simulink model "pmdc_speed_control"  (R2023a)
settings: Solver=FixedStepAuto  StartTime=0.0  StopTime=1.2  FixedStep=1e-5  RelTol=1e-3
values from neighbouring files (symbols this model uses):
  B = 0    [parabtl.m]    (also in pmdc_parameter.m; testpara.m)
  IaN = 62    [parabtl.m]    (also in pmdc_parameter.m = 25; testpara.m = 25)
  J = 0.05    [dcmotor_parameter.m]    (also in parabtl.m; pmdc_parameter.m = 0.00252; testpara.m = 0.00252)
  KE = (Ua - Ra*Ia)*9.55/n    (= 1.17113806452)    [dcmotor_parameter.m]    (also in parabtl.m; pmdc_parameter.m = 0.424975; testpara.m = 0.424975)
  Ki = Kp/Ti    [parabtl.m]    (also in pmdc_parameter.m)
  Kiv = Kpv/Tiv    [parabtl.m]    (also in pmdc_parameter.m)
  Kp = (Ra*Ta*OmegaN)/(2*Zeta)    [parabtl.m]    (also in pmdc_parameter.m)
  Kpv = TMech/(2*Teq)    [parabtl.m]    (also in pmdc_parameter.m)
  KT = KE    (= 1.17113806452)    [dcmotor_parameter.m]    (also in parabtl.m; pmdc_parameter.m = 0.424975; testpara.m = 0.424975)
  La = 5.2e-3    (= 0.0052)    [dcmotor_parameter.m]    (also in parabtl.m; pmdc_parameter.m = 0.0017; testpara.m = 0.0017)
  Ra = 0.32    [dcmotor_parameter.m]    (also in parabtl.m; pmdc_parameter.m = 0.26; testpara.m = 0.26)
  Td = 1/fsw    (= 0.0002)    [parabtl.m]    (also in pmdc_parameter.m)
  Tfi = 1/(5*fsw)    (= 4e-05)    [parabtl.m]    (also in pmdc_parameter.m)
  Tfv = 5*Tfi    (= 0.0002)    [parabtl.m]    (also in pmdc_parameter.m)
  UaN = 400    [parabtl.m]    (also in pmdc_parameter.m = 140; testpara.m = 140)
libraries: spsMosfetLib x12, spsDCVoltageSourceLib x3, simulink x3, spsVoltageMeasurementLib x3, spsDCMachineLib x2, sps_lib x1
settings Model: Creator=luand  LastModifiedBy=luand

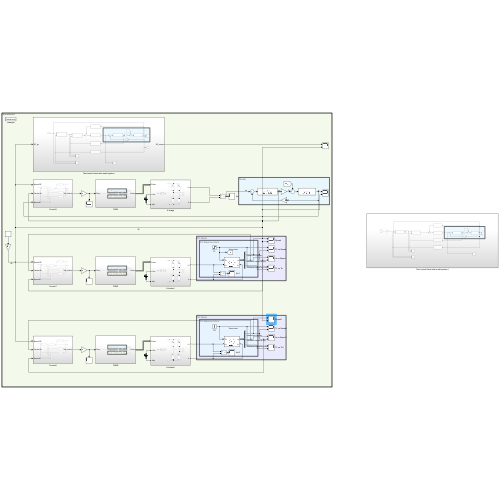
[thumbnail: Simulink's stored preview of the top-level diagram]
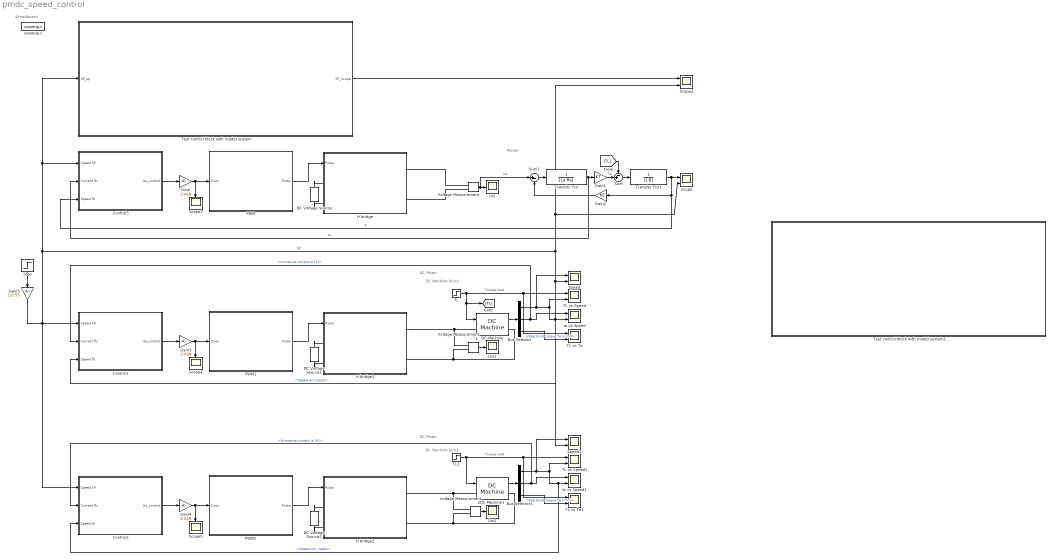
== system pmdc_speed_control ==
  note: Breadboard
  note: Model
  note: DC Motor
  note: DC Machine block
  note: DC Motor
  note: DC Machine block
  Bus Selector : BusSelector  OutputSignals=Speed wm (rad/s),Armature current ia (A),Electrical torque Te (n m)
  Bus Selector1 : BusSelector  OutputSignals=Speed wm (rad/s),Armature current ia (A),Electrical torque Te (n m)
  Control1 : Subsystem
  Control2 : Subsystem
  Control3 : Subsystem
  DC Machine : spsDCMachineLib/DC Machine  PresetModel=No  MechanicalLoad=Torque TL  FieldType=Permanent magnet  ShowDetailedParameters=on  MeasurementBus=off  RLa=[ Ra La ]  RLf="[ 240  120]"  Laf=1.8  MachineConstant=Torque constant (N.m/A)  Ke=1.8  Kt=KT  J=J  Bm=0  Tf=0  w0=0  Ifinit=1  TsPowergui=0  TsBlock=-1
  DC Machine1 : spsDCMachineLib/DC Machine  PresetModel=No  MechanicalLoad=Torque TL  FieldType=Permanent magnet  ShowDetailedParameters=on  MeasurementBus=off  RLa=[ Ra La ]  RLf="[ 240  120]"  Laf=1.8  MachineConstant=Torque constant (N.m/A)  Ke=1.8  Kt=KT  J=J  Bm=0  Tf=0  w0=0  Ifinit=1  TsPowergui=0  TsBlock=-1
  DC Voltage Source : spsDCVoltageSourceLib/DC Voltage Source  Amplitude=UaN  Measurements=None
  DC Voltage Source1 : spsDCVoltageSourceLib/DC Voltage Source  Amplitude=UaN  Measurements=None
  DC Voltage Source2 : spsDCVoltageSourceLib/DC Voltage Source  Amplitude=UaN  Measurements=None
  Gain : Gain  Gain=1/UaN
  Gain1 : Gain  Gain=KT
  Gain2 : Gain  Gain=KE
  Gain3 : Gain  Gain=1/UaN
  Gain4 : Gain  Gain=1/UaN
  Gain5 : Gain  Gain=1/9.55
  H bridge : Subsystem
  H bridge1 : Subsystem
  H bridge2 : Subsystem
  Ia vs Speed : Scope  NumInputPorts=2
  Ia vs Speed1 : Scope  NumInputPorts=2
  PWM : Subsystem
  PWM1 : Subsystem
  PWM2 : Subsystem
  Scope : Scope  NumInputPorts=2
  Scope2 : Scope  NumInputPorts=2
  Scope3 : Scope
  Scope4 : Scope
  Scope5 : Scope
  Speed : Scope  NumInputPorts=2
  Speed1 : Scope  NumInputPorts=2
  Step : Step  Time=.2  After=3000  SampleTime=0
  Sum : Sum  Inputs=-+|
  Sum1 : Sum  Inputs=|+-
  TL : Step  Time=0.3  After=0  SampleTime=0
  TL vs Speed : Scope  NumInputPorts=2
  TL vs Speed1 : Scope  NumInputPorts=2
  TL vs Te : Scope  NumInputPorts=2
  TL vs Te1 : Scope  NumInputPorts=2
  TL1 : Step  Time=0.3  After=0  SampleTime=0
  Test control block with model system : Subsystem
  Test control block with model system1 : Subsystem
  Transfer Fcn : TransferFcn  Denominator=[La Ra]
  Transfer Fcn1 : TransferFcn  Denominator=[J B]
  Uin : Scope
  Uin1 : Scope
  Uin2 : Scope
  Voltage Measurement : spsVoltageMeasurementLib/Voltage Measurement  PhasorSimulation=off  OutputType=Complex  PSBequivalent=0
  Voltage Measurement1 : spsVoltageMeasurementLib/Voltage Measurement  PhasorSimulation=off  OutputType=Complex  PSBequivalent=0
  Voltage Measurement2 : spsVoltageMeasurementLib/Voltage Measurement  PhasorSimulation=off  OutputType=Complex  PSBequivalent=0
  powergui : sps_lib/powergui  Priority=1  SimulationMode=Continuous  SampleTime=50e-6  frequency=60  Iterations=50  frequencyindice=0  Pbase=100e6  ErrMax=1e-4  UnitsV=kV  UnitsW=MW  buscounter=0  FunctionMessages=off  echomessages=off  EnableUseOfTLC=off  CurrentSourceSwitches=off  DisableSnubberDevices=off  DisableRonSwitches=off  DisableVfSwitches=off  DisplayEquations=off  AutomaticDiscreteSolvers=off  SolverType=Tustin/Backward Euler (TBE)  Interpol=off  ExternalGateDelay=off  methode=off  Ts=100  x0status=blocks  SPID=on  SwTol=0  HookPort=off  NonlinearTolerance=1e-4  nMaxIteration=100  ContinueOnMaxIteration=off  RestoreLinks=warning  ResistiveCurrentMeasurement=off  Frange=[0:2:500]  Ylog=off  Xlog=on  ShowGrid=off  save=off  variable=ZData  structure=0  ZoomFFT=off  StartTime=0.0  cycles=1  DisplayStyle=1  fundamental=60  FreqAxis=off  MaxFrequency=1000  frequencyindicesteady=1  RmsSteady=1  display=off
  wires:
  DC Machine/1 -> Bus Selector/1
  Bus Selector/2 -> Ia vs Speed/1, Control1/2(Current fb)  "<Armature current ia (A)>"
  Bus Selector/3 -> TL vs Te/2  "<Electrical torque Te (n m)>"
  Bus Selector/1 -> Speed/1, TL vs Speed/2, Control1/3(Speed fb), Ia vs Speed/2  "<Speed wm (rad/s)>"
  TL/1 -> DC Machine/1, [TL], TL vs Te/1, TL vs Speed/1  "Torque load"
  Control3/1(Ua_control) -> Gain/1
  PWM/1(Pulse) -> H bridge/1(Pulse)
  Voltage Measurement1/1 -> Uin1/1
  Voltage Measurement2/1 -> Uin2/1
  TL1/1 -> TL vs Speed1/1, TL vs Te1/1, DC Machine1/1  "Torque load"
  Bus Selector1/1 -> Control2/3(Speed fb), Ia vs Speed1/2, TL vs Speed1/2, Speed1/1  "<Speed wm (rad/s)>"
  Bus Selector1/3 -> TL vs Te1/2  "<Electrical torque Te (n m)>"
  Bus Selector1/2 -> Control2/2(Current fb), Ia vs Speed1/1  "<Armature current ia (A)>"
  DC Machine1/1 -> Bus Selector1/1
  Transfer Fcn/1 -> Control3/2(Current fb), Gain1/1  "Ia"
  Sum/1 -> Transfer Fcn1/1
  Sum1/1 -> Transfer Fcn/1
  Transfer Fcn1/1 -> Gain2/1, Control3/3(Speed fb), Scope/1  "w"
  Gain1/1 -> Sum/2  "Te"
  [TL] -> Sum/1
  Gain2/1 -> Sum1/2
  Voltage Measurement/1 -> Sum1/1, Uin/1  "Ua"
  Control1/1(Ua_control) -> Gain3/1
  PWM2/1(Pulse) -> H bridge2/1(Pulse)
  PWM1/1(Pulse) -> H bridge1/1(Pulse)
  Gain3/1 -> PWM1/1(Duty), Scope4/1
  Step/1 -> Gain5/1
  Gain5/1 -> Scope2/2, Scope/2, Speed/2, Speed1/2, Test control block with model system/1(SP_sp), Control3/1(Speed SP), Control2/1(Speed SP), Control1/1(Speed SP)  "SP"
  Control2/1(Ua_control) -> Gain4/1
  Gain4/1 -> PWM2/1(Duty), Scope5/1
  Test control block with model system/1(SP_scope) -> Scope2/1
  Gain/1 -> Scope3/1, PWM/1(Duty)
  connections:
  Voltage Measurement2/LConn2 -- DC Machine1/RConn1 -- H bridge2/RConn2
  Voltage Measurement2/LConn1 -- H bridge2/RConn1 -- DC Machine1/LConn1
  Voltage Measurement1/LConn2 -- H bridge1/RConn2 -- DC Machine/RConn1
  DC Voltage Source/RConn1 -- H bridge/LConn1
  DC Voltage Source/LConn1 -- H bridge/LConn2
  DC Voltage Source1/LConn1 -- H bridge1/LConn2
  DC Voltage Source1/RConn1 -- H bridge1/LConn1
  DC Voltage Source2/RConn1 -- H bridge2/LConn1
  DC Voltage Source2/LConn1 -- H bridge2/LConn2
  H bridge1/RConn1 -- DC Machine/LConn1 -- Voltage Measurement1/LConn1
  Voltage Measurement/LConn1 -- H bridge/RConn1
  Voltage Measurement/LConn2 -- H bridge/RConn2

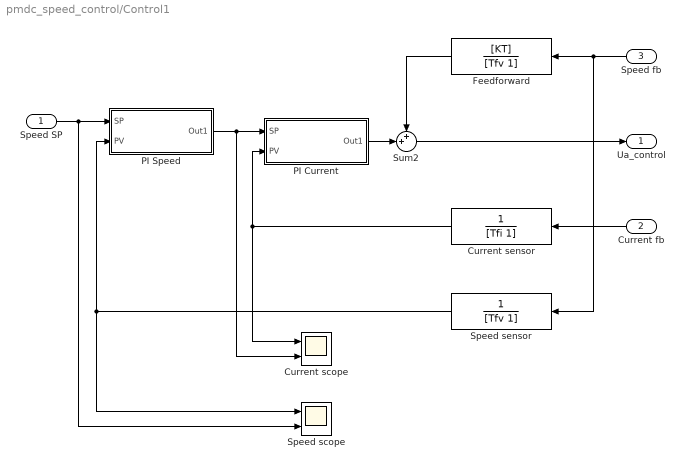
== system pmdc_speed_control/Control1 ==
  Speed SP : Inport
  Current fb : Inport  Port=2
  Speed fb : Inport  Port=3
  Current scope : Scope  NumInputPorts=2
  Current sensor : TransferFcn  Denominator=[Tfi 1]
  Feedforward : TransferFcn  Numerator=[KT]  Denominator=[Tfv 1]
  PI Current : Subsystem
  PI Speed : Subsystem
  Speed scope : Scope  NumInputPorts=2
  Speed sensor : TransferFcn  Denominator=[Tfv 1]
  Sum2 : Sum  Inputs=++|
  Ua_control : Outport
  wires:
  Speed SP/1 -> PI Speed/1(SP), Speed scope/2
  Speed sensor/1 -> Speed scope/1, PI Speed/2(PV)
  Sum2/1 -> Ua_control/1
  PI Current/1(Out1) -> Sum2/2
  Feedforward/1 -> Sum2/1
  Current sensor/1 -> PI Current/2(PV), Current scope/1
  PI Speed/1(Out1) -> PI Current/1(SP), Current scope/2
  Speed fb/1 -> Speed sensor/1, Feedforward/1
  Current fb/1 -> Current sensor/1

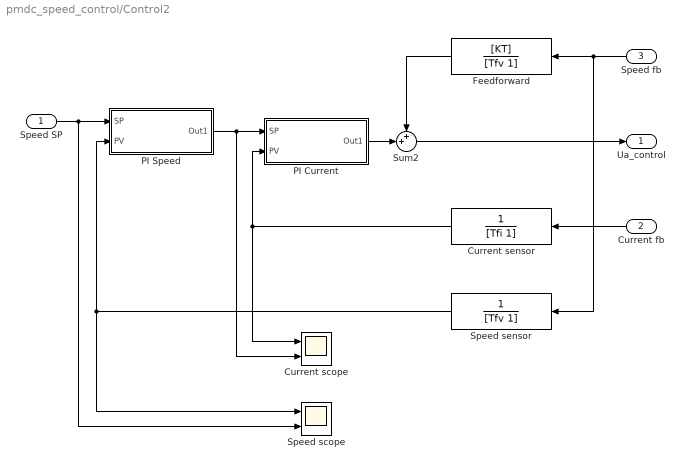
== system pmdc_speed_control/Control2 ==
  Speed SP : Inport
  Current fb : Inport  Port=2
  Speed fb : Inport  Port=3
  Current scope : Scope  NumInputPorts=2
  Current sensor : TransferFcn  Denominator=[Tfi 1]
  Feedforward : TransferFcn  Numerator=[KT]  Denominator=[Tfv 1]
  PI Current : Subsystem
  PI Speed : Subsystem
  Speed scope : Scope  NumInputPorts=2
  Speed sensor : TransferFcn  Denominator=[Tfv 1]
  Sum2 : Sum  Inputs=++|
  Ua_control : Outport
  wires:
  Current fb/1 -> Current sensor/1
  Speed fb/1 -> Feedforward/1, Speed sensor/1
  PI Speed/1(Out1) -> Current scope/2, PI Current/1(SP)
  Current sensor/1 -> Current scope/1, PI Current/2(PV)
  Feedforward/1 -> Sum2/1
  PI Current/1(Out1) -> Sum2/2
  Sum2/1 -> Ua_control/1
  Speed sensor/1 -> PI Speed/2(PV), Speed scope/1
  Speed SP/1 -> Speed scope/2, PI Speed/1(SP)

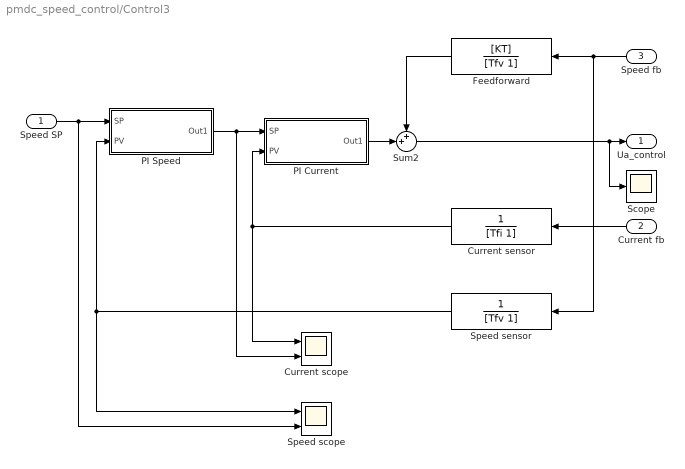
== system pmdc_speed_control/Control3 ==
  Speed SP : Inport
  Current fb : Inport  Port=2
  Speed fb : Inport  Port=3
  Current scope : Scope  NumInputPorts=2
  Current sensor : TransferFcn  Denominator=[Tfi 1]
  Feedforward : TransferFcn  Numerator=[KT]  Denominator=[Tfv 1]
  PI Current : Subsystem
  PI Speed : Subsystem
  Scope : Scope
  Speed scope : Scope  NumInputPorts=2
  Speed sensor : TransferFcn  Denominator=[Tfv 1]
  Sum2 : Sum  Inputs=++|
  Ua_control : Outport
  wires:
  Current fb/1 -> Current sensor/1
  Speed fb/1 -> Feedforward/1, Speed sensor/1
  PI Speed/1(Out1) -> Current scope/2, PI Current/1(SP)
  Current sensor/1 -> Current scope/1, PI Current/2(PV)
  Feedforward/1 -> Sum2/1
  PI Current/1(Out1) -> Sum2/2
  Sum2/1 -> Scope/1, Ua_control/1
  Speed sensor/1 -> PI Speed/2(PV), Speed scope/1
  Speed SP/1 -> Speed scope/2, PI Speed/1(SP)

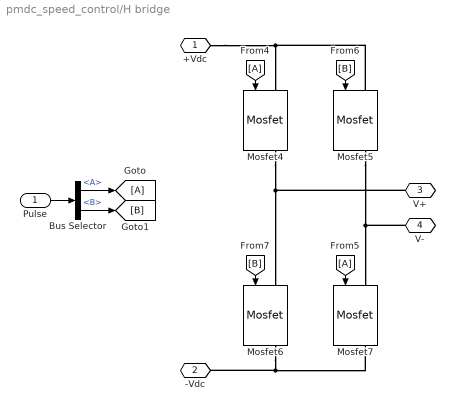
== system pmdc_speed_control/H bridge ==
  Pulse : Inport
  Bus Selector : BusSelector  OutputSignals=A,B
  From4 : From
  From5 : From
  Goto : Goto
  Mosfet{4..7} (4 alike) : spsMosfetLib/Mosfet  Ron=0.1  Lon=0  Rd=0.01  Vfd=0  IC=0  Rs=1e5  Cs=inf  Measurements=on
  +Vdc : PMIOPort  Side=Left
  -Vdc : PMIOPort  Port=2  Side=Left
  V+ : PMIOPort  Port=3  Side=Right
  V- : PMIOPort  Port=4  Side=Right
  wires:
  Pulse/1 -> Bus Selector/1
  Bus Selector/1 -> Goto/1  "<A>"
  Bus Selector/2 -> [B]  "<B>"
  From5/1 -> Mosfet7/1
  [B] -> Mosfet6/1
  [B] -> Mosfet5/1
  From4/1 -> Mosfet4/1
  connections:
  Mosfet4/RConn1 -- V+/RConn1 -- Mosfet6/LConn1
  Mosfet7/RConn1 -- Mosfet6/RConn1 -- -Vdc/RConn1
  Mosfet5/LConn1 -- +Vdc/RConn1 -- Mosfet4/LConn1
  Mosfet5/RConn1 -- V-/RConn1 -- Mosfet7/LConn1

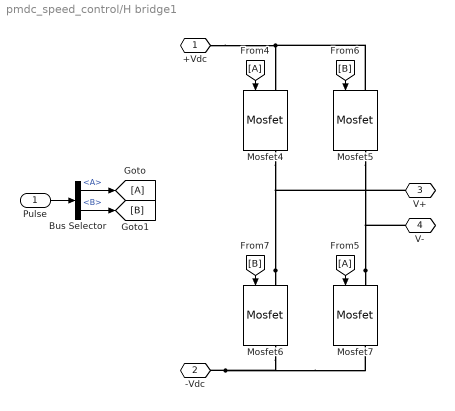
== system pmdc_speed_control/H bridge1 ==
  Pulse : Inport
  Bus Selector : BusSelector  OutputSignals=A,B
  From4 : From
  From5 : From
  Goto : Goto
  Mosfet{4..7} (4 alike) : spsMosfetLib/Mosfet  Ron=0.1  Lon=0  Rd=0.01  Vfd=0  IC=0  Rs=1e5  Cs=inf  Measurements=on
  +Vdc : PMIOPort  Side=Left
  -Vdc : PMIOPort  Port=2  Side=Left
  V+ : PMIOPort  Port=3  Side=Right
  V- : PMIOPort  Port=4  Side=Right
  wires:
  From4/1 -> Mosfet4/1
  [B] -> Mosfet5/1
  [B] -> Mosfet6/1
  From5/1 -> Mosfet7/1
  Bus Selector/2 -> [B]  "<B>"
  Bus Selector/1 -> Goto/1  "<A>"
  Pulse/1 -> Bus Selector/1
  connections:
  Mosfet7/LConn1 -- V-/RConn1 -- Mosfet5/RConn1
  +Vdc/RConn1 -- Mosfet4/LConn1 -- Mosfet5/LConn1
  -Vdc/RConn1 -- Mosfet7/RConn1 -- Mosfet6/RConn1
  Mosfet6/LConn1 -- V+/RConn1 -- Mosfet4/RConn1

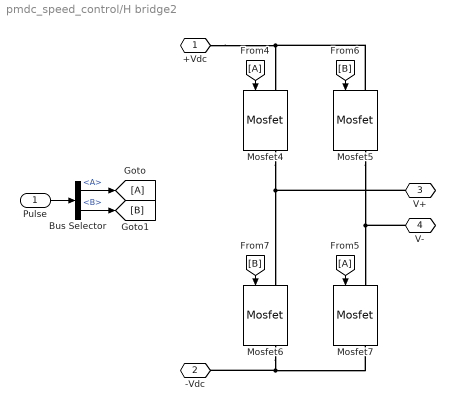
== system pmdc_speed_control/H bridge2 ==
  Pulse : Inport
  Bus Selector : BusSelector  OutputSignals=A,B
  From4 : From
  From5 : From
  Goto : Goto
  Mosfet{4..7} (4 alike) : spsMosfetLib/Mosfet  Ron=0.1  Lon=0  Rd=0.01  Vfd=0  IC=0  Rs=1e5  Cs=inf  Measurements=on
  +Vdc : PMIOPort  Side=Left
  -Vdc : PMIOPort  Port=2  Side=Left
  V+ : PMIOPort  Port=3  Side=Right
  V- : PMIOPort  Port=4  Side=Right
  wires:
  Pulse/1 -> Bus Selector/1
  Bus Selector/1 -> Goto/1  "<A>"
  Bus Selector/2 -> [B]  "<B>"
  From5/1 -> Mosfet7/1
  [B] -> Mosfet6/1
  [B] -> Mosfet5/1
  From4/1 -> Mosfet4/1
  connections:
  Mosfet4/RConn1 -- V+/RConn1 -- Mosfet6/LConn1
  Mosfet6/RConn1 -- Mosfet7/RConn1 -- -Vdc/RConn1
  Mosfet5/LConn1 -- Mosfet4/LConn1 -- +Vdc/RConn1
  Mosfet5/RConn1 -- V-/RConn1 -- Mosfet7/LConn1

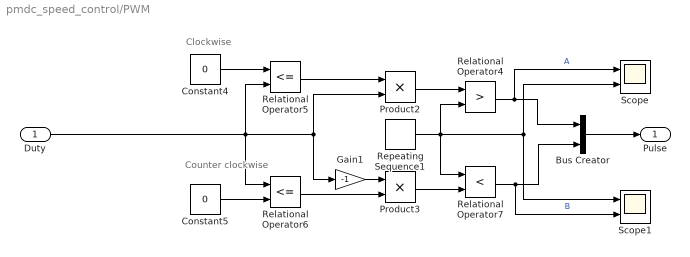
== system pmdc_speed_control/PWM ==
  note: Counter clockwise
  note: Clockwise
  Duty : Inport
  Bus Creator : BusCreator  Inputs=2
  Constant4 : Constant  Value=0
  Constant5 : Constant  Value=0
  Gain1 : Gain  Gain=-1
  Product2 : Product
  Product3 : Product
  Relational Operator4 : RelationalOperator  Operator=>  OutDataTypeStr=boolean  RndMeth=Simplest  InputSameDT=off
  Relational Operator5 : RelationalOperator  Operator=<=  OutDataTypeStr=boolean  RndMeth=Simplest  InputSameDT=off
  Relational Operator6 : RelationalOperator  Operator=<=  OutDataTypeStr=boolean  RndMeth=Simplest  InputSameDT=off
  Relational Operator7 : RelationalOperator  Operator=<  OutDataTypeStr=boolean  RndMeth=Simplest  InputSameDT=off
  Repeating Sequence1 : simulink/Sources/Repeating Sequence  rep_seq_t=[0 1e-3]  rep_seq_y=[0 1]
  Scope : Scope  NumInputPorts=2
  Scope1 : Scope  NumInputPorts=2
  Pulse : Outport
  wires:
  Bus Creator/1 -> Pulse/1
  Relational Operator6/1 -> Product3/2
  Repeating Sequence1/1 -> Scope1/1, Scope/2, Relational Operator7/1, Relational Operator4/2
  Duty/1 -> Product2/2, Gain1/1, Relational Operator5/2, Relational Operator6/1
  Relational Operator5/1 -> Product2/1
  Constant5/1 -> Relational Operator6/2
  Product3/1 -> Relational Operator7/2
  Gain1/1 -> Product3/1
  Constant4/1 -> Relational Operator5/1
  Relational Operator7/1 -> Scope1/2, Bus Creator/2  "B"
  Relational Operator4/1 -> Bus Creator/1, Scope/1  "A"
  Product2/1 -> Relational Operator4/1

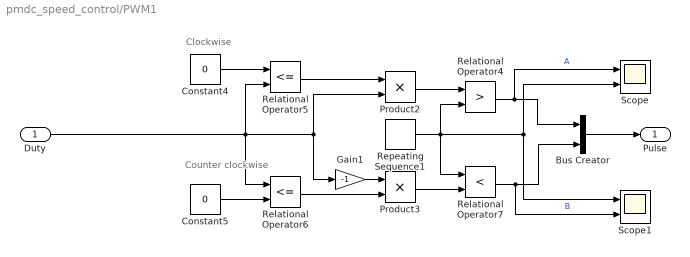
== system pmdc_speed_control/PWM1 ==
  note: Clockwise
  note: Counter clockwise
  Duty : Inport
  Bus Creator : BusCreator  Inputs=2
  Constant4 : Constant  Value=0
  Constant5 : Constant  Value=0
  Gain1 : Gain  Gain=-1
  Product2 : Product
  Product3 : Product
  Relational Operator4 : RelationalOperator  Operator=>  OutDataTypeStr=boolean  RndMeth=Simplest  InputSameDT=off
  Relational Operator5 : RelationalOperator  Operator=<=  OutDataTypeStr=boolean  RndMeth=Simplest  InputSameDT=off
  Relational Operator6 : RelationalOperator  Operator=<=  OutDataTypeStr=boolean  RndMeth=Simplest  InputSameDT=off
  Relational Operator7 : RelationalOperator  Operator=<  OutDataTypeStr=boolean  RndMeth=Simplest  InputSameDT=off
  Repeating Sequence1 : simulink/Sources/Repeating Sequence  rep_seq_t=[0 1e-3]  rep_seq_y=[0 1]
  Scope : Scope  NumInputPorts=2
  Scope1 : Scope  NumInputPorts=2
  Pulse : Outport
  wires:
  Product2/1 -> Relational Operator4/1
  Relational Operator4/1 -> Scope/1, Bus Creator/1  "A"
  Relational Operator7/1 -> Bus Creator/2, Scope1/2  "B"
  Constant4/1 -> Relational Operator5/1
  Gain1/1 -> Product3/1
  Product3/1 -> Relational Operator7/2
  Constant5/1 -> Relational Operator6/2
  Relational Operator5/1 -> Product2/1
  Duty/1 -> Relational Operator6/1, Gain1/1, Product2/2, Relational Operator5/2
  Repeating Sequence1/1 -> Relational Operator4/2, Relational Operator7/1, Scope/2, Scope1/1
  Relational Operator6/1 -> Product3/2
  Bus Creator/1 -> Pulse/1

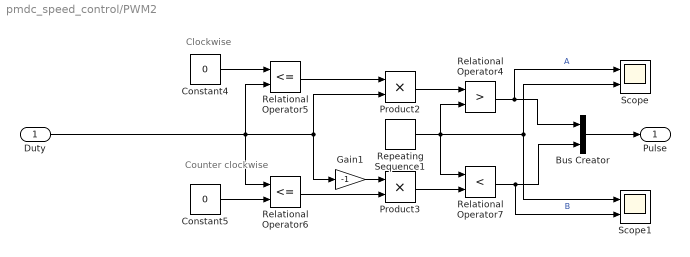
== system pmdc_speed_control/PWM2 ==
  note: Counter clockwise
  note: Clockwise
  Duty : Inport
  Bus Creator : BusCreator  Inputs=2
  Constant4 : Constant  Value=0
  Constant5 : Constant  Value=0
  Gain1 : Gain  Gain=-1
  Product2 : Product
  Product3 : Product
  Relational Operator4 : RelationalOperator  Operator=>  OutDataTypeStr=boolean  RndMeth=Simplest  InputSameDT=off
  Relational Operator5 : RelationalOperator  Operator=<=  OutDataTypeStr=boolean  RndMeth=Simplest  InputSameDT=off
  Relational Operator6 : RelationalOperator  Operator=<=  OutDataTypeStr=boolean  RndMeth=Simplest  InputSameDT=off
  Relational Operator7 : RelationalOperator  Operator=<  OutDataTypeStr=boolean  RndMeth=Simplest  InputSameDT=off
  Repeating Sequence1 : simulink/Sources/Repeating Sequence  rep_seq_t=[0 1e-3]  rep_seq_y=[0 1]
  Scope : Scope  NumInputPorts=2
  Scope1 : Scope  NumInputPorts=2
  Pulse : Outport
  wires:
  Bus Creator/1 -> Pulse/1
  Relational Operator6/1 -> Product3/2
  Repeating Sequence1/1 -> Scope1/1, Scope/2, Relational Operator7/1, Relational Operator4/2
  Duty/1 -> Relational Operator5/2, Product2/2, Gain1/1, Relational Operator6/1
  Relational Operator5/1 -> Product2/1
  Constant5/1 -> Relational Operator6/2
  Product3/1 -> Relational Operator7/2
  Gain1/1 -> Product3/1
  Constant4/1 -> Relational Operator5/1
  Relational Operator7/1 -> Scope1/2, Bus Creator/2  "B"
  Relational Operator4/1 -> Bus Creator/1, Scope/1  "A"
  Product2/1 -> Relational Operator4/1

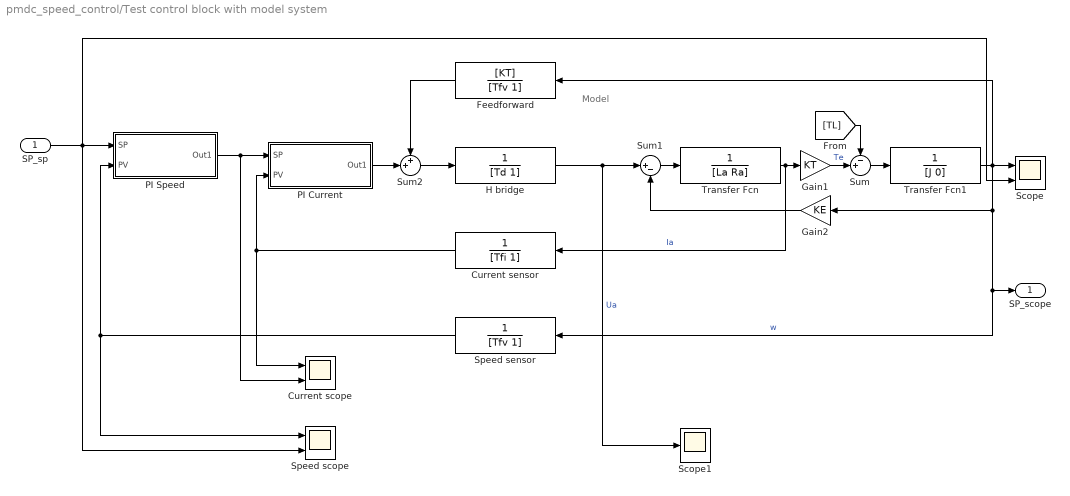
== system pmdc_speed_control/Test control block with model system ==
  note: Model
  SP_sp : Inport
  Current scope : Scope  NumInputPorts=2
  Current sensor : TransferFcn  Denominator=[Tfi 1]
  Feedforward : TransferFcn  Numerator=[KT]  Denominator=[Tfv 1]
  Gain1 : Gain  Gain=KT
  Gain2 : Gain  Gain=KE
  H bridge : TransferFcn  Denominator=[Td 1]
  PI Current : Subsystem
  PI Speed : Subsystem
  Scope : Scope  NumInputPorts=2
  Scope1 : Scope
  Speed scope : Scope  NumInputPorts=2
  Speed sensor : TransferFcn  Denominator=[Tfv 1]
  Sum : Sum  Inputs=-+|
  Sum1 : Sum  Inputs=|+-
  Sum2 : Sum  Inputs=++|
  Transfer Fcn : TransferFcn  Denominator=[La Ra]
  Transfer Fcn1 : TransferFcn  Denominator=[J 0]
  SP_scope : Outport
  wires:
  PI Speed/1(Out1) -> Current scope/2, PI Current/1(SP)
  SP_sp/1 -> Speed scope/2, Scope/2, PI Speed/1(SP)
  H bridge/1 -> Scope1/1, Sum1/1  "Ua"
  PI Current/1(Out1) -> Sum2/2
  Transfer Fcn1/1 -> Feedforward/1, Scope/1, Speed sensor/1, SP_scope/1, Gain2/1  "w"
  Sum1/1 -> Transfer Fcn/1
  Gain2/1 -> Sum1/2
  Transfer Fcn/1 -> Current sensor/1, Gain1/1  "Ia"
  Sum2/1 -> H bridge/1
  Feedforward/1 -> Sum2/1
  Current sensor/1 -> Current scope/1, PI Current/2(PV)
  Gain1/1 -> Sum/2  "Te"
  [TL] -> Sum/1
  Speed sensor/1 -> PI Speed/2(PV), Speed scope/1
  Sum/1 -> Transfer Fcn1/1

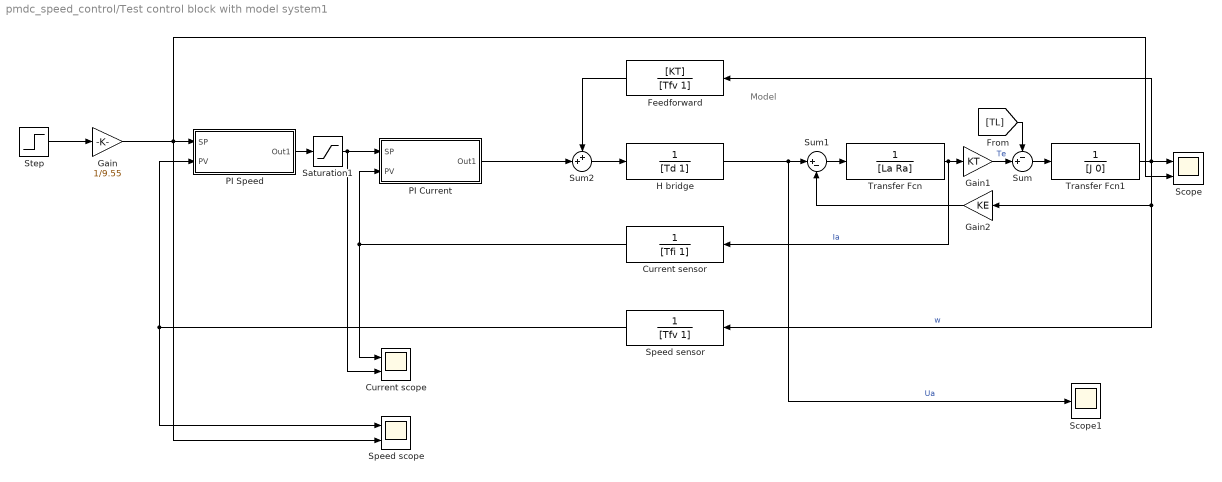
== system pmdc_speed_control/Test control block with model system1 ==
  note: Model
  Current scope : Scope  NumInputPorts=2
  Current sensor : TransferFcn  Denominator=[Tfi 1]
  Feedforward : TransferFcn  Numerator=[KT]  Denominator=[Tfv 1]
  Gain : Gain  Gain=1/9.55
  Gain1 : Gain  Gain=KT
  Gain2 : Gain  Gain=KE
  H bridge : TransferFcn  Denominator=[Td 1]
  PI Current : Subsystem
  PI Speed : Subsystem
  Saturation1 : Saturate  UpperLimit=6*IaN  LowerLimit=-6*IaN
  Scope : Scope  NumInputPorts=2
  Scope1 : Scope
  Speed scope : Scope  NumInputPorts=2
  Speed sensor : TransferFcn  Denominator=[Tfv 1]
  Step : Step  Time=.2  After=3000  SampleTime=0
  Sum : Sum  Inputs=-+|
  Sum1 : Sum  Inputs=|+-
  Sum2 : Sum  Inputs=++|
  Transfer Fcn : TransferFcn  Denominator=[La Ra]
  Transfer Fcn1 : TransferFcn  Denominator=[J 0]
  wires:
  Step/1 -> Gain/1
  PI Current/1(Out1) -> Sum2/2
  Transfer Fcn1/1 -> Feedforward/1, Scope/1, Speed sensor/1, Gain2/1  "w"
  Sum1/1 -> Transfer Fcn/1
  Gain2/1 -> Sum1/2
  Transfer Fcn/1 -> Current sensor/1, Gain1/1  "Ia"
  Sum2/1 -> H bridge/1
  Feedforward/1 -> Sum2/1
  Current sensor/1 -> PI Current/2(PV), Current scope/1
  Gain1/1 -> Sum/2  "Te"
  [TL] -> Sum/1
  Speed sensor/1 -> Speed scope/1, PI Speed/2(PV)
  Sum/1 -> Transfer Fcn1/1
  Gain/1 -> PI Speed/1(SP), Scope/2, Speed scope/2
  H bridge/1 -> Scope1/1, Sum1/1  "Ua"
  PI Speed/1(Out1) -> Saturation1/1
  Saturation1/1 -> Current scope/2, PI Current/1(SP)

== system pmdc_speed_control/Control1/PI Current ==
  SP : Inport
  PV : Inport  Port=2
  Gain : Gain  Gain=Kp
  Gain1 : Gain  Gain=Ki
  Scope : Scope  NumInputPorts=2
  Sum : Sum  Inputs=|+-
  Sum1 : Sum  Inputs=|++
  Transfer Fcn : TransferFcn  Denominator=[1 0]
  Out1 : Outport
  wires:
  SP/1 -> Scope/1, Sum/1
  PV/1 -> Sum/2, Scope/2
  Sum/1 -> Gain1/1, Gain/1
  Gain1/1 -> Transfer Fcn/1
  Gain/1 -> Sum1/1
  Transfer Fcn/1 -> Sum1/2
  Sum1/1 -> Out1/1

== system pmdc_speed_control/Control1/PI Speed ==
  SP : Inport
  PV : Inport  Port=2
  Gain : Gain  Gain=Kpv
  Gain1 : Gain  Gain=Kiv
  Scope : Scope  NumInputPorts=2
  Sum : Sum  Inputs=|+-
  Sum1 : Sum  Inputs=|++
  Transfer Fcn : TransferFcn  Denominator=[1 0]
  Out1 : Outport
  wires:
  Sum1/1 -> Out1/1
  Transfer Fcn/1 -> Sum1/2
  Gain/1 -> Sum1/1
  Gain1/1 -> Transfer Fcn/1
  Sum/1 -> Gain/1, Gain1/1
  PV/1 -> Scope/2, Sum/2
  SP/1 -> Sum/1, Scope/1

== system pmdc_speed_control/Control2/PI Current ==
  SP : Inport
  PV : Inport  Port=2
  Gain : Gain  Gain=Kp
  Gain1 : Gain  Gain=Ki
  Scope : Scope  NumInputPorts=2
  Sum : Sum  Inputs=|+-
  Sum1 : Sum  Inputs=|++
  Transfer Fcn : TransferFcn  Denominator=[1 0]
  Out1 : Outport
  wires:
  Sum1/1 -> Out1/1
  Transfer Fcn/1 -> Sum1/2
  Gain/1 -> Sum1/1
  Gain1/1 -> Transfer Fcn/1
  Sum/1 -> Gain/1, Gain1/1
  PV/1 -> Scope/2, Sum/2
  SP/1 -> Sum/1, Scope/1

== system pmdc_speed_control/Control2/PI Speed ==
  SP : Inport
  PV : Inport  Port=2
  Gain : Gain  Gain=Kpv
  Gain1 : Gain  Gain=Kiv
  Scope : Scope  NumInputPorts=2
  Sum : Sum  Inputs=|+-
  Sum1 : Sum  Inputs=|++
  Transfer Fcn : TransferFcn  Denominator=[1 0]
  Out1 : Outport
  wires:
  SP/1 -> Scope/1, Sum/1
  PV/1 -> Sum/2, Scope/2
  Sum/1 -> Gain1/1, Gain/1
  Gain1/1 -> Transfer Fcn/1
  Gain/1 -> Sum1/1
  Transfer Fcn/1 -> Sum1/2
  Sum1/1 -> Out1/1

== system pmdc_speed_control/Control3/PI Current ==
  SP : Inport
  PV : Inport  Port=2
  Gain : Gain  Gain=Kp
  Gain1 : Gain  Gain=Ki
  Scope : Scope  NumInputPorts=2
  Sum : Sum  Inputs=|+-
  Sum1 : Sum  Inputs=|++
  Transfer Fcn : TransferFcn  Denominator=[1 0]
  Out1 : Outport
  wires:
  Sum1/1 -> Out1/1
  Transfer Fcn/1 -> Sum1/2
  Gain/1 -> Sum1/1
  Gain1/1 -> Transfer Fcn/1
  Sum/1 -> Gain/1, Gain1/1
  PV/1 -> Scope/2, Sum/2
  SP/1 -> Sum/1, Scope/1

== system pmdc_speed_control/Control3/PI Speed ==
  SP : Inport
  PV : Inport  Port=2
  Gain : Gain  Gain=Kpv
  Gain1 : Gain  Gain=Kiv
  Scope : Scope  NumInputPorts=2
  Sum : Sum  Inputs=|+-
  Sum1 : Sum  Inputs=|++
  Transfer Fcn : TransferFcn  Denominator=[1 0]
  Out1 : Outport
  wires:
  SP/1 -> Scope/1, Sum/1
  PV/1 -> Sum/2, Scope/2
  Sum/1 -> Gain1/1, Gain/1
  Gain1/1 -> Transfer Fcn/1
  Gain/1 -> Sum1/1
  Transfer Fcn/1 -> Sum1/2
  Sum1/1 -> Out1/1

== system pmdc_speed_control/Test control block with model system/PI Current ==
  SP : Inport
  PV : Inport  Port=2
  Gain : Gain  Gain=Kp
  Gain1 : Gain  Gain=Ki
  Scope : Scope  NumInputPorts=2
  Sum : Sum  Inputs=|+-
  Sum1 : Sum  Inputs=|++
  Transfer Fcn : TransferFcn  Denominator=[1 0]
  Out1 : Outport
  wires:
  Sum1/1 -> Out1/1
  Transfer Fcn/1 -> Sum1/2
  Gain/1 -> Sum1/1
  Gain1/1 -> Transfer Fcn/1
  Sum/1 -> Gain/1, Gain1/1
  PV/1 -> Scope/2, Sum/2
  SP/1 -> Sum/1, Scope/1

== system pmdc_speed_control/Test control block with model system/PI Speed ==
  SP : Inport
  PV : Inport  Port=2
  Gain : Gain  Gain=Kpv
  Gain1 : Gain  Gain=Kiv
  Scope : Scope  NumInputPorts=2
  Sum : Sum  Inputs=|+-
  Sum1 : Sum  Inputs=|++
  Transfer Fcn : TransferFcn  Denominator=[1 0]
  Out1 : Outport
  wires:
  SP/1 -> Scope/1, Sum/1
  PV/1 -> Sum/2, Scope/2
  Sum/1 -> Gain1/1, Gain/1
  Gain1/1 -> Transfer Fcn/1
  Gain/1 -> Sum1/1
  Transfer Fcn/1 -> Sum1/2
  Sum1/1 -> Out1/1

== system pmdc_speed_control/Test control block with model system1/PI Current ==
  SP : Inport
  PV : Inport  Port=2
  Gain : Gain  Gain=Kp
  Gain1 : Gain  Gain=Ki
  Scope : Scope  NumInputPorts=2
  Sum : Sum  Inputs=|+-
  Sum1 : Sum  Inputs=|++
  Transfer Fcn : TransferFcn  Denominator=[1 0]
  Out1 : Outport
  wires:
  Sum1/1 -> Out1/1
  Transfer Fcn/1 -> Sum1/2
  Gain/1 -> Sum1/1
  Gain1/1 -> Transfer Fcn/1
  Sum/1 -> Gain/1, Gain1/1
  PV/1 -> Scope/2, Sum/2
  SP/1 -> Sum/1, Scope/1

== system pmdc_speed_control/Test control block with model system1/PI Speed ==
  SP : Inport
  PV : Inport  Port=2
  Gain : Gain  Gain=Kpv
  Gain1 : Gain  Gain=Kiv
  Scope : Scope  NumInputPorts=2
  Sum : Sum  Inputs=|+-
  Sum1 : Sum  Inputs=|++
  Transfer Fcn : TransferFcn  Denominator=[1 0]
  Out1 : Outport
  wires:
  SP/1 -> Scope/1, Sum/1
  PV/1 -> Sum/2, Scope/2
  Sum/1 -> Gain1/1, Gain/1
  Gain1/1 -> Transfer Fcn/1
  Gain/1 -> Sum1/1
  Transfer Fcn/1 -> Sum1/2
  Sum1/1 -> Out1/1
